simulink model "atrias_boom_nmSt_kinSw_v3"  (R2015a)
settings: Solver=ode23t  StartTime=0.0  StopTime=t_end  FixedStep=0.001  MaxStep=1e-3  RelTol=1e-3
InitFcn:
  | addpath('../common/')
  | colors
StartFcn:
  | tic
StopFcn:
  | %stopscript
values from neighbouring files (symbols this model uses):
  dt_a_dTrunk_boom = 5    [main_1_nmSt_kinSw.m]    (also in main_2_nmSt_kinSw_v2.m; main_3_nmSt_kinSw_v3.m; main_4_nmSt_kinSw_v4.m)
  dt_fade_boomCtrl = 2    [main_1_nmSt_kinSw.m]    (also in main_2_nmSt_kinSw_v2.m; main_3_nmSt_kinSw_v3.m; main_4_nmSt_kinSw_v4.m)
  initial_boom_yaw = 15*pi/180    (= 0.261799387799)    [main_2_nmSt_kinSw_v2.m]    (also in main_3_nmSt_kinSw_v3.m; main_4_nmSt_kinSw_v4.m)
  kd_boom_roll_Ctrl = 0    [main_1_nmSt_kinSw - Copy.m]    (also in main_1_nmSt_kinSw.m; main_2_nmSt_kinSw_v2.m; main_3_nmSt_kinSw_v3.m; main_4_nmSt_kinSw_v4.m)
  kd_boom_yaw_Ctrl = 0.1*kp_boom_yaw_Ctrl    (= 100000000)    [main_1_nmSt_kinSw - Copy.m]    (also in main_1_nmSt_kinSw.m = 1000000000; main_2_nmSt_kinSw_v2.m = 10000000; main_3_nmSt_kinSw_v3.m = 10000000; main_4_nmSt_kinSw_v4.m = 10000000)
  kd_motor = 0.90*2*sqrt(3.75*kp_motor)    [main_1_nmSt_kinSw - Copy.m]
  kinSw_alpha_start = 100*pi/180    (= 1.74532925199)    [main_1_nmSt_kinSw - Copy.m]    (also in main_1_nmSt_kinSw.m = 1.91986217719; main_2_nmSt_kinSw_v2.m = 1.83259571459; main_3_nmSt_kinSw_v3.m = 1.83259571459; main_4_nmSt_kinSw_v4.m = 1.83259571459)
  kinSw_alpha_tgt = 80*pi/180    (= 1.3962634016)    [main_1_nmSt_kinSw - Copy.m]    (also in main_1_nmSt_kinSw.m = 1.2217304764; main_2_nmSt_kinSw_v2.m = 1.2217304764; main_3_nmSt_kinSw_v3.m = 1.2217304764; main_4_nmSt_kinSw_v4.m = 1.2217304764)
  kinSw_t_start = 1.5    [main_1_nmSt_kinSw - Copy.m]    (also in main_1_nmSt_kinSw.m; main_2_nmSt_kinSw_v2.m = 0.5; main_3_nmSt_kinSw_v3.m = 0.5; main_4_nmSt_kinSw_v4.m = 0.5)
  kp_boom_roll_Ctrl = 0    [main_1_nmSt_kinSw - Copy.m]    (also in main_1_nmSt_kinSw.m; main_2_nmSt_kinSw_v2.m; main_3_nmSt_kinSw_v3.m; main_4_nmSt_kinSw_v4.m)
  kp_boom_yaw_Ctrl = 1e9    (= 1000000000)    [main_1_nmSt_kinSw - Copy.m]    (also in main_1_nmSt_kinSw.m = 10000000000; main_2_nmSt_kinSw_v2.m = 100000000; main_3_nmSt_kinSw_v3.m = 100000000; main_4_nmSt_kinSw_v4.m = 100000000)
  kp_motor = 3000    [main_1_nmSt_kinSw - Copy.m]
  max_back_bar_angle = 262.4*pi/180    (= 4.57974395723)    [main_1_nmSt_kinSw - Copy.m]
  max_front_bar_angle = 194.8*pi/180    (= 3.39990138288)    [main_1_nmSt_kinSw - Copy.m]
  min_back_bar_angle = 165.0*pi/180    (= 2.87979326579)    [main_1_nmSt_kinSw - Copy.m]
  min_front_bar_angle = 98.0*pi/180    (= 1.71042266695)    [main_1_nmSt_kinSw - Copy.m]
  poser_LLegAlp = (initial_l_leg_angle -pi/2)*180/pi    (= 105)    [main_2_nmSt_kinSw_v2.m]    (also in main_3_nmSt_kinSw_v3.m; main_4_nmSt_kinSw_v4.m)
  poser_LLegLen = initial_l_leg_length    (= 0.88)    [main_2_nmSt_kinSw_v2.m]    (also in main_3_nmSt_kinSw_v3.m; main_4_nmSt_kinSw_v4.m)
  poser_RLegAlp = (initial_r_leg_angle -pi/2)*180/pi    (= 75)    [main_2_nmSt_kinSw_v2.m]    (also in main_3_nmSt_kinSw_v3.m; main_4_nmSt_kinSw_v4.m)
  poser_RLegLen = initial_r_leg_length    (= 0.9)    [main_2_nmSt_kinSw_v2.m]    (also in main_3_nmSt_kinSw_v3.m; main_4_nmSt_kinSw_v4.m)
  tEnd_boomCtrl = t_end    (= 20)    [main_1_nmSt_kinSw - Copy.m]    (also in main_1_nmSt_kinSw.m = 3; main_2_nmSt_kinSw_v2.m = 7.5; main_3_nmSt_kinSw_v3.m = 7.5; main_4_nmSt_kinSw_v4.m = 7.5)
  tStart_boomCtrl = 1    [main_1_nmSt_kinSw - Copy.m]    (also in main_1_nmSt_kinSw.m = 0; main_2_nmSt_kinSw_v2.m = 0.5; main_3_nmSt_kinSw_v3.m = 0.5; main_4_nmSt_kinSw_v4.m = 0.5)
  tune_kinSw_alpha_start = kinSw_alpha_start*180/pi    (= 105)    [main_2_nmSt_kinSw_v2.m]    (also in main_3_nmSt_kinSw_v3.m; main_4_nmSt_kinSw_v4.m)
  tune_kinSw_alpha_tgt = kinSw_alpha_tgt*180/pi    (= 70)    [main_2_nmSt_kinSw_v2.m]    (also in main_3_nmSt_kinSw_v3.m; main_4_nmSt_kinSw_v4.m)
  tune_kinSw_len_min = kinSw_lclr    (= 0.7)    [main_2_nmSt_kinSw_v2.m]    (also in main_3_nmSt_kinSw_v3.m = 0.6)
  tune_kinSw_len_tgt = kinSw_len_tgt    (= 0.9)    [main_2_nmSt_kinSw_v2.m]    (also in main_3_nmSt_kinSw_v3.m)
  tune_M1_G = St_FGain_VAS*FmaxVAS    [main_2_nmSt_kinSw_v2.m]    (also in main_3_nmSt_kinSw_v3.m; main_4_nmSt_kinSw_v4.m)
  tune_M3_0 = CtrlPar_theta0*180/pi    [main_2_nmSt_kinSw_v2.m]    (also in main_3_nmSt_kinSw_v3.m; main_4_nmSt_kinSw_v4.m)
  tune_M3_D = St_GainDTh_HFL    [main_2_nmSt_kinSw_v2.m]    (also in main_3_nmSt_kinSw_v3.m; main_4_nmSt_kinSw_v4.m)
  tune_M3_P = St_GainTh_HFL    [main_2_nmSt_kinSw_v2.m]    (also in main_3_nmSt_kinSw_v3.m; main_4_nmSt_kinSw_v4.m)
  tune_M4_G = 1    [main_3_nmSt_kinSw_v3.m]    (also in main_4_nmSt_kinSw_v4.m)
  v_dTrunk_boom = 1.3    [main_1_nmSt_kinSw.m]    (also in main_2_nmSt_kinSw_v2.m; main_3_nmSt_kinSw_v3.m; main_4_nmSt_kinSw_v4.m)
undefined symbols (not defined in the file or in its folder): A1_notch_f1, A2_notch_f1, A_lpf_dtau, A_lpf_velocity, ankle_stiffness, B1_lpf_dtau, B1_lpf_velocity, B1_notch_f1, B2_lpf_dtau, B2_lpf_velocity, B2_notch_f1, b_hmotor, b_leg_spring, b_rotor, base_color_d, boom_color_d, boom_mount_to_center_diagonal, breakaway_friction, c_jointstop, contactThr, coulomb_friction, d_com, delta_phi_max, delta_phi_max_buffer, delta_phi_max_dropoff, delta_phi_min, fblink_color_d, floor_color_d, FmaxBFSH, FmaxGLU, FmaxHAM, FmaxHFL, FmaxRF, FmaxVAS, foot_color_d, FPCtrlPar, friction_linear_zone, g, gain_nodes_sea_torque, HIP_MTR_MAX_CONT_TORQUE, HIP_MTR_MAX_TORQUE, hshaft_color_d, initial_boom_pitch, initial_boom_roll, initial_hip_roll, initial_winch_angle, j_motor, k_gn, k_gt, k_leg_spring, K_notch_f1, k_phi, k_sea, Kb_leg, kd_lateral, kd_shin_max, kd_shin_min, kd_splay_max, kd_splay_min, kd_thigh_max ... (+186)
libraries: sm_lib x210, nesl_utility x140, simulink x65, simulink_extras x32, fl_lib x16, mblibv1 x2, commnoisgen2 x1
(part 6 of 17)

== system atrias_boom_nmSt_kinSw_v3/Mechanical System Layer/Ground Contact Models/flat ground (LHeel) ==
  Cnt : Inport
  Constant : Constant  Value=0
  Constant1 : Constant  Value=[0 0 1]
  Mux4 : Mux  Inputs=5
  Selector25 : Selector  InputPortWidth=3
  Selector26 : Selector  InputPortWidth=7  Indices=[1 2 3 6 4 5 7]
  Selector27 : Selector  InputPortWidth=3  Indices=3
  Env : Outport
  wires:
  Mux4/1 -> Selector26/1
  Constant1/1 -> Mux4/3
  Cnt/1 -> Selector27/1, Selector25/1
  Selector27/1 -> Mux4/4
  Constant/1 -> Mux4/5, Mux4/1
  Selector25/1 -> Mux4/2
  Selector26/1 -> Env/1

== system atrias_boom_nmSt_kinSw_v3/Mechanical System Layer/Ground Contact Models/flat ground (RBall) ==
  Cnt : Inport
  Constant : Constant  Value=0
  Constant1 : Constant  Value=[0 0 1]
  Mux4 : Mux  Inputs=5
  Selector25 : Selector  InputPortWidth=3
  Selector26 : Selector  InputPortWidth=7  Indices=[1 2 3 6 4 5 7]
  Selector27 : Selector  InputPortWidth=3  Indices=3
  Env : Outport
  wires:
  Mux4/1 -> Selector26/1
  Constant1/1 -> Mux4/3
  Cnt/1 -> Selector27/1, Selector25/1
  Selector27/1 -> Mux4/4
  Constant/1 -> Mux4/5, Mux4/1
  Selector25/1 -> Mux4/2
  Selector26/1 -> Env/1

== system atrias_boom_nmSt_kinSw_v3/Mechanical System Layer/Ground Contact Models/flat ground (RHeel) ==
  Cnt : Inport
  Constant : Constant  Value=0
  Constant1 : Constant  Value=[0 0 1]
  Mux4 : Mux  Inputs=5
  Selector25 : Selector  InputPortWidth=3
  Selector26 : Selector  InputPortWidth=7  Indices=[1 2 3 6 4 5 7]
  Selector27 : Selector  InputPortWidth=3  Indices=3
  Env : Outport
  wires:
  Mux4/1 -> Selector26/1
  Constant1/1 -> Mux4/3
  Cnt/1 -> Selector27/1, Selector25/1
  Selector27/1 -> Mux4/4
  Constant/1 -> Mux4/5, Mux4/1
  Selector25/1 -> Mux4/2
  Selector26/1 -> Env/1

== system atrias_boom_nmSt_kinSw_v3/Mechanical System Layer/L Hip Shaft/Frame Data ==
  Kinematic Data : ToWorkspace  VariableName=l_hip_out  SampleTime=output_sample_time
      settings: Save2DSignal=2-D array (concatenate along first dimension)
  Mux : Mux
  PS-Simulink Converter{,1..3} (4 alike) : nesl_utility/PS-Simulink Converter  PhysicalDomain=network_engine_domain  SubClassName=ps_output  LeftPortType=input  RightPortType=output  PseudoPeriodic=off  Frequencies=[]  Unit=1  AffineConversion=off
  Transform Sensor : sm_lib/Frames and Transforms/Transform Sensor  MeasurementFrame=World  SenseAngle=off  SenseAxis=off  SenseAngle1=off  SenseAngle2=off  SenseAngle3=off  SenseQ=on  SenseR=off  SenseOmegaX=off  SenseOmegaY=off  SenseOmegaZ=off  SenseOmega1=off  SenseOmega2=off  SenseOmega3=off  SenseQDot=off  SenseRDot=off  SenseAlphaX=off  SenseAlphaY=off  SenseAlphaZ=off  SenseAlpha1=off  SenseAlpha2=off  SenseAlpha3=off  SenseQDDot=off  SenseRDDot=off  SenseX=on  SenseY=on  SenseZ=on  SenseRad=off  SenseAzim=off  SenseDist=off  SenseInc=off  SenseXDot=off  SenseYDot=off  SenseZDot=off  SenseRadDot=off  SenseAzimDot=off  SenseDistDot=off  SenseIncDot=off  SenseXDDot=off  SenseYDDot=off  SenseZDDot=off  SenseRadDDot=off  SenseAzimDDot=off  SenseDistDDot=off  SenseIncDDot=off  BlockFunction=simmechanics.library.frames_transforms.transform_sensor
  World Frame : sm_lib/Frames and Transforms/World Frame  BlockFunction=simmechanics.library.frames_transforms.world_frame
  Frame : PMIOPort  Port=1  Side=Left
  wires:
  Mux/1 -> Kinematic Data/1
  PS-Simulink Converter/1 -> Mux/1
  PS-Simulink Converter1/1 -> Mux/2
  PS-Simulink Converter2/1 -> Mux/3
  PS-Simulink Converter3/1 -> Mux/4
  connections:
  PS-Simulink Converter3/LConn1 -- Transform Sensor/RConn5
  PS-Simulink Converter2/LConn1 -- Transform Sensor/RConn4
  PS-Simulink Converter1/LConn1 -- Transform Sensor/RConn3
  PS-Simulink Converter/LConn1 -- Transform Sensor/RConn2
  Transform Sensor/RConn1 -- Frame/RConn1
  Transform Sensor/LConn1 -- World Frame/RConn1

== system atrias_boom_nmSt_kinSw_v3/Mechanical System Layer/L Leg/Angle Range Map ==
  "[-pi, pi]" : Inport
  Constant : Constant  Value=2*pi
  Sum3 : Sum  Inputs=|++
  Switch : Switch  ZeroCross=off
  "[0,2*pi]" : Outport
  wires:
  "[-pi, pi]"/1 -> Sum3/1, Switch/1, Switch/2
  Sum3/1 -> Switch/3
  Constant/1 -> Sum3/2
  Switch/1 -> "[0,2*pi]"/1

== system atrias_boom_nmSt_kinSw_v3/Mechanical System Layer/L Leg/Angle Range Map1 ==
  "[-pi, pi]" : Inport
  Constant : Constant  Value=2*pi
  Sum3 : Sum  Inputs=|++
  Switch : Switch  ZeroCross=off
  "[0,2*pi]" : Outport
  wires:
  Switch/1 -> "[0,2*pi]"/1
  Constant/1 -> Sum3/2
  Sum3/1 -> Switch/3
  "[-pi, pi]"/1 -> Switch/2, Switch/1, Sum3/1

== system atrias_boom_nmSt_kinSw_v3/Mechanical System Layer/L Leg/Four Bar Link ==
  CS1 to CS2 : sm_lib/Frames and Transforms/Rigid Transform  TranslationMethod=Cartesian  TranslationLengthUnit=m  TranslationStandardAxis=+Z  TranslationStandardOffset=0  TranslationCartesianOffset=[0 -l_seg 0]  TranslationROffset=0  TranslationROffsetUnits=m  TranslationZOffset=0  TranslationZOffsetUnits=m  TranslationThetaOffset=0  TranslationThetaOffsetUnits=deg  RotationMethod=None  RotationAngleUnits=deg  RotationStandardAxis=+Z  RotationAngle=0  RotationArbitraryAxis=[0 0 1]  FollAlignAxisA=+X  BaseAlignAxisA=+Y  FollAlignAxisB=+Y  BaseAlignAxisB=+Z  RotationMatrix=[1 0 0; 0 1 0; 0 0 1]  BlockFunction=simmechanics.library.frames_transforms.rigid_transform
  Frame Data : Subsystem
  Solid : sm_lib/Body Elements/Solid  InertiaType=Custom  Mass=m_fblink  MassUnits=kg  CenterOfMass=com_fblink  CenterOfMassUnits=m  MomentsOfInertia=i_fblink_moments  MomentsOfInertiaUnits=kg*m^2  ProductsOfInertia=i_fblink_products  ProductsOfInertiaUnits=kg*m^2  DensityBased=on  Density=1000  DensityUnits=kg/(m^3)  GraphicType=FromGeometry  MarkerShape=Sphere  MarkerSize=10  MarkerSizeUnits=m  GraphicVisPropType=AdvancedVisualProperties  GraphicDiffuseColor=fblink_color_d  GraphicSpecularColor=[0.5 0.5 0.5 1.0]  GraphicAmbientColor=[fblink_color_d*0.5 1.0]  GraphicEmissiveColor=[0.0 0.0 0.0 1.0]  GraphicShininess=128  GraphicOpacity=1.0  GeometryShape=FromFile  RectangleSize=[1 1]  RectangleSizeUnits=m  BrickDimensions=[0.1 l_seg 0.1]  BrickDimensionUnits=m  CylinderRadius=l_rad  CylinderRadiusUnits=m  CylinderLength=l_seg  CylinderLengthUnits=m  SphereRadius=1  SphereRadiusUnits=m  EllipsoidRadii=[1 1 1]  EllipsoidRadiiUnits=m  ExtrusionCrossSection=[1 1; -1 1; -1 -1; 1 -1]  ExtrusionCrossSectionUnits=m  ExtrusionLength=1  ExtrusionLengthUnits=m  PolygonNumSides=3  PolygonOuterRadius=1  PolygonOuterRadiusUnits=m  ExtGeomFileType=STL  ExtGeomFileName=../models/four_bar_link.stl  ExtGeomFileUnits=m  RevolutionCrossSection=[1 1; 1 -1; 2 -1; 2 1]  RevolutionCrossSectionUnits=m  RevolutionExtent=Full  RevolutionAngle=180  RevolutionAngleUnits=deg  BlockFunction=simmechanics.library.body_elements.solid
  CS1 : PMIOPort  Port=1  Side=Left
  CS2 : PMIOPort  Port=2  Side=Right
  connections:
  CS2/RConn1 -- CS1 to CS2/RConn1
  Solid/RConn1 -- CS1/RConn1 -- Frame Data/LConn1 -- CS1 to CS2/LConn1

== system atrias_boom_nmSt_kinSw_v3/Mechanical System Layer/L Leg/Lower Leg ==
  CS1 to CS2 : sm_lib/Frames and Transforms/Rigid Transform  TranslationMethod=Cartesian  TranslationLengthUnit=m  TranslationStandardAxis=+Z  TranslationStandardOffset=0  TranslationCartesianOffset=[0 -lowerleg_12 0]  TranslationROffset=0  TranslationROffsetUnits=m  TranslationZOffset=0  TranslationZOffsetUnits=m  TranslationThetaOffset=0  TranslationThetaOffsetUnits=deg  RotationMethod=None  RotationAngleUnits=deg  RotationStandardAxis=+Z  RotationAngle=0  RotationArbitraryAxis=[0 0 1]  FollAlignAxisA=+X  BaseAlignAxisA=+Y  FollAlignAxisB=+Y  BaseAlignAxisB=+Z  RotationMatrix=[1 0 0; 0 1 0; 0 0 1]  BlockFunction=simmechanics.library.frames_transforms.rigid_transform
  CS1 to CS3 : sm_lib/Frames and Transforms/Rigid Transform  TranslationMethod=Cartesian  TranslationLengthUnit=m  TranslationStandardAxis=+Z  TranslationStandardOffset=0  TranslationCartesianOffset=[0 -l_seg 0]  TranslationROffset=0  TranslationROffsetUnits=m  TranslationZOffset=0  TranslationZOffsetUnits=m  TranslationThetaOffset=0  TranslationThetaOffsetUnits=deg  RotationMethod=None  RotationAngleUnits=deg  RotationStandardAxis=+Z  RotationAngle=0  RotationArbitraryAxis=[0 0 1]  FollAlignAxisA=+X  BaseAlignAxisA=+Y  FollAlignAxisB=+Y  BaseAlignAxisB=+Z  RotationMatrix=[1 0 0; 0 1 0; 0 0 1]  BlockFunction=simmechanics.library.frames_transforms.rigid_transform
  Frame Data : Subsystem
  Solid : sm_lib/Body Elements/Solid  InertiaType=Custom  Mass=m_lowerleg  MassUnits=kg  CenterOfMass=com_lowerleg  CenterOfMassUnits=m  MomentsOfInertia=i_lowerleg_moments  MomentsOfInertiaUnits=kg*m^2  ProductsOfInertia=i_lowerleg_products  ProductsOfInertiaUnits=kg*m^2  DensityBased=on  Density=1000  DensityUnits=kg/(m^3)  GraphicType=FromGeometry  MarkerShape=Sphere  MarkerSize=10  MarkerSizeUnits=m  GraphicVisPropType=AdvancedVisualProperties  GraphicDiffuseColor=lowerleg_color_d  GraphicSpecularColor=[0.5 0.5 0.5 1.0]  GraphicAmbientColor=[lowerleg_color_d*0.5 1.0]  GraphicEmissiveColor=[0.0 0.0 0.0 1.0]  GraphicShininess=128  GraphicOpacity=1.0  GeometryShape=FromFile  RectangleSize=[1 1]  RectangleSizeUnits=m  BrickDimensions=[0.1 l_seg 0.1]  BrickDimensionUnits=m  CylinderRadius=l_rad  CylinderRadiusUnits=m  CylinderLength=l_seg  CylinderLengthUnits=m  SphereRadius=1  SphereRadiusUnits=m  EllipsoidRadii=[1 1 1]  EllipsoidRadiiUnits=m  ExtrusionCrossSection=[1 1; -1 1; -1 -1; 1 -1]  ExtrusionCrossSectionUnits=m  ExtrusionLength=1  ExtrusionLengthUnits=m  PolygonNumSides=3  PolygonOuterRadius=1  PolygonOuterRadiusUnits=m  ExtGeomFileType=STL  ExtGeomFileName=../models/lower_leg.STL  ExtGeomFileUnits=m  RevolutionCrossSection=[1 1; 1 -1; 2 -1; 2 1]  RevolutionCrossSectionUnits=m  RevolutionExtent=Full  RevolutionAngle=180  RevolutionAngleUnits=deg  BlockFunction=simmechanics.library.body_elements.solid
  CS1 : PMIOPort  Port=1  Side=Left
  CS2 : PMIOPort  Port=2  Side=Right
  CS3 : PMIOPort  Port=3  Side=Right
  connections:
  CS3/RConn1 -- CS1 to CS3/RConn1
  Frame Data/LConn1 -- CS1 to CS3/LConn1 -- CS1 to CS2/LConn1 -- Solid/RConn1 -- CS1/RConn1
  CS2/RConn1 -- CS1 to CS2/RConn1

== system atrias_boom_nmSt_kinSw_v3/Mechanical System Layer/L Leg/Mechanical Limits ==
  note: Thigh-Shin Flexion Collision
  note: Thigh-Shin Collision
  note: Mechanical Limits Model
  dphi_shin : Inport
  phi_shin : Inport  Port=2
  dphi_thigh : Inport  Port=3
  phi_thigh : Inport  Port=4
  Compare To Constant5 : simulink/Logic and Bit Operations/Compare To Constant  relop=<=  const=phi_max_collision  OutDataTypeStr=boolean  ZeroCross=off
  Compare To Zero{,1..5} (6 alike) : simulink/Logic and Bit Operations/Compare To Zero  relop=<=  OutDataTypeStr=boolean  ZeroCross=off
  Constant : Constant  Value=delta_phi_min
  Constant1 : Constant  Value=phi_shin_max
  Constant2 : Constant  Value=phi_thigh_min
  Constant3 : Constant  Value=delta_phi_max
  Constant4 : Constant  Value=phi_shin_min
  Constant5 : Constant  Value=phi_thigh_max
  Enabled Subsystem : Subsystem  TreatAsAtomicUnit=on
  Gain : Gain  Gain=-1
  Gain1 : Gain  Gain=-1
  Gain2 : Gain  Gain=-1
  Logical Operator : Logic  Operator=OR  Inputs=1  AllPortsSameDT=off  OutDataTypeStr=boolean
  Mux : Mux  Inputs=6
  Shin Max Collision Model : Subsystem
  Shin Min Collision Model : Subsystem
  Stop Simulation6 : Stop
  Sum{1..3,5,7} (5 alike) : Sum  Inputs=-+|
  Sum10 : Sum  Inputs=+-|
  Sum11 : Sum  Inputs=-|+
  Sum4 : Sum  Inputs=+-|
  Sum6 : Sum  Inputs=+|-
  Sum8 : Sum  Inputs=+-|
  Sum9 : Sum  Inputs=-|+
  Thigh Max Collision Model : Subsystem
  Thigh Min Collision Model : Subsystem
  Thigh-Shin Collision Model : Subsystem
  Thigh-Shin Collision Model1 : Subsystem
  tau_shin_col : Outport
  tau_thigh_shin_col : Outport  Port=2
  tau_thigh_col : Outport  Port=3
  wires:
  Compare To Constant5/1 -> Logical Operator/1, Enabled Subsystem/1(Col_Flags)
  Sum4/1 -> Shin Max Collision Model/1(phi [rad]), Compare To Zero1/1, [col_r_shin_max]
  Sum10/1 -> [col_r_thigh_max], Compare To Zero5/1, Thigh Max Collision Model/1(phi [rad])
  Logical Operator/1 -> Enabled Subsystem/Enable, Stop Simulation6/1
  Mux/1 -> Compare To Constant5/1
  [col_r_leg_flexion] -> Mux/6
  [col_r_leg_extension] -> Mux/5
  [col_r_shin_min] -> Mux/4
  [col_r_shin_max] -> Mux/3
  [col_r_thigh_min] -> Mux/2
  [col_r_thigh_max] -> Mux/1
  Thigh Max Collision Model/1(tau_interaction[Nm]) -> Sum11/1
  Gain1/1 -> Thigh Max Collision Model/2(vphi [rad/s])
  Thigh Min Collision Model/1(tau_interaction[Nm]) -> Sum11/2
  Sum11/1 -> tau_thigh_col/1
  Compare To Zero5/1 -> Thigh Max Collision Model/Enable
  Constant5/1 -> Sum10/1
  Sum6/1 -> tau_thigh_shin_col/1
  Shin Min Collision Model/1(tau_interaction[Nm]) -> Sum9/2
  Shin Max Collision Model/1(tau_interaction[Nm]) -> Sum9/1
  Sum9/1 -> tau_shin_col/1
  dphi_shin/1 -> Shin Min Collision Model/2(vphi [rad/s]), Gain/1, Sum2/2
  Sum7/1 -> Shin Min Collision Model/1(phi [rad]), Compare To Zero4/1, [col_r_shin_min]
  Constant4/1 -> Sum7/1
  Compare To Zero4/1 -> Shin Min Collision Model/Enable
  Gain2/1 -> Thigh-Shin Collision Model1/2(vphi [rad/s])
  Thigh-Shin Collision Model1/1(tau_interaction[Nm]) -> Sum6/2
  Thigh-Shin Collision Model/1(tau_interaction[Nm]) -> Sum6/1
  Sum8/1 -> Thigh-Shin Collision Model1/1(delta_phi [rad]), Compare To Zero3/1, [col_r_leg_flexion]
  Constant3/1 -> Sum8/1
  Compare To Zero3/1 -> Thigh-Shin Collision Model1/Enable
  Compare To Zero2/1 -> Thigh Min Collision Model/Enable
  Gain/1 -> Shin Max Collision Model/2(vphi [rad/s])
  Sum5/1 -> Thigh Min Collision Model/1(phi [rad]), Compare To Zero2/1, [col_r_thigh_min]
  Constant2/1 -> Sum5/1
  dphi_thigh/1 -> Sum2/1, Gain1/1, Thigh Min Collision Model/2(vphi [rad/s])
  phi_thigh/1 -> Sum1/1, Sum5/2, Sum10/2
  Constant1/1 -> Sum4/1
  Compare To Zero1/1 -> Shin Max Collision Model/Enable
  Sum3/1 -> Thigh-Shin Collision Model/1(delta_phi [rad]), Compare To Zero/1, [col_r_leg_extension]
  Constant/1 -> Sum3/1
  Sum2/1 -> Thigh-Shin Collision Model/2(vphi [rad/s]), Gain2/1
  phi_shin/1 -> Sum4/2, Sum7/2, Sum1/2
  Sum1/1 -> Sum3/2, Sum8/2
  Compare To Zero/1 -> Thigh-Shin Collision Model/Enable

== system atrias_boom_nmSt_kinSw_v3/Mechanical System Layer/L Leg/Shin ==
  CS1 to CS2 : sm_lib/Frames and Transforms/Rigid Transform  TranslationMethod=Cartesian  TranslationLengthUnit=m  TranslationStandardAxis=+Z  TranslationStandardOffset=0  TranslationCartesianOffset=[0 -shin_12 0]  TranslationROffset=0  TranslationROffsetUnits=m  TranslationZOffset=0  TranslationZOffsetUnits=m  TranslationThetaOffset=0  TranslationThetaOffsetUnits=deg  RotationMethod=None  RotationAngleUnits=deg  RotationStandardAxis=+Z  RotationAngle=0  RotationArbitraryAxis=[0 0 1]  FollAlignAxisA=+X  BaseAlignAxisA=+Y  FollAlignAxisB=+Y  BaseAlignAxisB=+Z  RotationMatrix=[1 0 0; 0 1 0; 0 0 1]  BlockFunction=simmechanics.library.frames_transforms.rigid_transform
  Frame Data : Subsystem
  Solid : sm_lib/Body Elements/Solid  InertiaType=Custom  Mass=m_shin  MassUnits=kg  CenterOfMass=com_shin  CenterOfMassUnits=m  MomentsOfInertia=i_shin_moments  MomentsOfInertiaUnits=kg*m^2  ProductsOfInertia=i_shin_products  ProductsOfInertiaUnits=kg*m^2  DensityBased=on  Density=1000  DensityUnits=kg/(m^3)  GraphicType=FromGeometry  MarkerShape=Sphere  MarkerSize=10  MarkerSizeUnits=m  GraphicVisPropType=AdvancedVisualProperties  GraphicDiffuseColor=shin_color_d  GraphicSpecularColor=[0.5 0.5 0.5 1.0]  GraphicAmbientColor=[shin_color_d*0.5 1.0]  GraphicEmissiveColor=[0.0 0.0 0.0 1.0]  GraphicShininess=128  GraphicOpacity=1.0  GeometryShape=FromFile  RectangleSize=[1 1]  RectangleSizeUnits=m  BrickDimensions=[1 1 1]  BrickDimensionUnits=m  CylinderRadius=l_rad  CylinderRadiusUnits=m  CylinderLength=l_seg  CylinderLengthUnits=m  SphereRadius=1  SphereRadiusUnits=m  EllipsoidRadii=[1 1 1]  EllipsoidRadiiUnits=m  ExtrusionCrossSection=[1 1; -1 1; -1 -1; 1 -1]  ExtrusionCrossSectionUnits=m  ExtrusionLength=1  ExtrusionLengthUnits=m  PolygonNumSides=3  PolygonOuterRadius=1  PolygonOuterRadiusUnits=m  ExtGeomFileType=STL  ExtGeomFileName=../models/shin.STL  ExtGeomFileUnits=m  RevolutionCrossSection=[1 1; 1 -1; 2 -1; 2 1]  RevolutionCrossSectionUnits=m  RevolutionExtent=Full  RevolutionAngle=180  RevolutionAngleUnits=deg  BlockFunction=simmechanics.library.body_elements.solid
  CS1 : PMIOPort  Port=1  Side=Left
  CS2 : PMIOPort  Port=2  Side=Right
  connections:
  CS1 to CS2/LConn1 -- CS1/RConn1 -- Frame Data/LConn1 -- Solid/RConn1
  CS2/RConn1 -- CS1 to CS2/RConn1

== system atrias_boom_nmSt_kinSw_v3/Mechanical System Layer/L Leg/Shin SEA ==
  note: Shin SEA Mechanics
  Shin Gear Torque [Nm] : Inport
  Shin Joint [rad rad/s] : Inport  Port=2
  Demux : Demux  Outputs=2
  Gain : Gain  Gain=k_leg_spring
  Gain1 : Gain  Gain=b_leg_spring
  Initial Gear Angle : Constant  Value=shin_initial_l
  Inverse Gear Ratio2 : Gain  Gain=1/N
  Inverse Gear Ratio3 : Gain  Gain=Kt_leg
  Inverse Gear Ratio4 : Gain  Gain=1/Kt_leg
  Motor Efficiency : Gain  Gain=mu_motor
  Motor Controller : Subsystem  Commented=on
  Motor Electromagnetism : Subsystem  Commented=on
  Rotor Damping : Gain  Gain=b_rotor
  Rotor and Gearing : Subsystem
  Sum : Sum  Inputs=++|
  Sum2 : Sum  Inputs=+|-
  Sum3 : Sum  Inputs=|+-
  Sum4 : Sum  Inputs=+|-
  Sum5 : Sum  Inputs=|++
  Torque Limiter (outside) 2 : Saturate  UpperLimit=LEG_MTR_MAX_TORQUE  LowerLimit=-LEG_MTR_MAX_TORQUE  ZeroCross=off
      settings: AttributesFormatString=Hi: %<UpperLimit>\nLo: %<LowerLimit>
  Rotor Joint Conn : PMIOPort  Port=1  Side=Left
  Shin Joint Torque [Nm] : Outport
  Shin Gear [rad] : Outport  Port=2
  wires:
  Sum2/1 -> Gain/1
  Sum5/1 -> Rotor and Gearing/2(Spring Torque [Nm]), Shin Joint Torque [Nm]/1
  Sum3/1 -> Motor Efficiency/1
  Rotor Damping/1 -> Sum3/2
  Gain/1 -> Sum5/1  "tau_load"
  Gain1/1 -> Sum5/2
  Sum4/1 -> Gain1/1
  Shin Joint [rad rad/s]/1 -> Demux/1
  Demux/1 -> Sum2/2
  Demux/2 -> Sum4/2
  Inverse Gear Ratio3/1 -> Sum3/1
  Initial Gear Angle/1 -> Sum/1
  Sum/1 -> Shin Gear [rad]/1, Sum2/1
  Rotor and Gearing/1(Gearhead Position [rad]) -> Sum/2
  Rotor and Gearing/2(Gearhead Velocity [rad/s]) -> Sum4/1
  Motor Efficiency/1 -> Rotor and Gearing/1(Rotor Torque [Nm])
  Inverse Gear Ratio4/1 -> Inverse Gear Ratio3/1
  Motor Controller/1(Voltage [V]) -> Motor Electromagnetism/1(Voltage [V])
  Motor Electromagnetism/1(Current [A]) -> Motor Controller/2(Measured Current [A])
  Shin Gear Torque [Nm]/1 -> Torque Limiter (outside) 2/1
  Inverse Gear Ratio2/1 -> Inverse Gear Ratio4/1
  Rotor and Gearing/3(Rotor Velocity [rad/s]) -> Rotor Damping/1
  Torque Limiter (outside) 2/1 -> Inverse Gear Ratio2/1
  connections:
  Rotor and Gearing/LConn1 -- Rotor Joint Conn/RConn1

== system atrias_boom_nmSt_kinSw_v3/Mechanical System Layer/L Leg/Thigh ==
  CS1 to CS2 : sm_lib/Frames and Transforms/Rigid Transform  TranslationMethod=Cartesian  TranslationLengthUnit=m  TranslationStandardAxis=+Z  TranslationStandardOffset=0  TranslationCartesianOffset=[0 -l_seg 0]  TranslationROffset=0  TranslationROffsetUnits=m  TranslationZOffset=0  TranslationZOffsetUnits=m  TranslationThetaOffset=0  TranslationThetaOffsetUnits=deg  RotationMethod=None  RotationAngleUnits=deg  RotationStandardAxis=+Z  RotationAngle=0  RotationArbitraryAxis=[0 0 1]  FollAlignAxisA=+X  BaseAlignAxisA=+Y  FollAlignAxisB=+Y  BaseAlignAxisB=+Z  RotationMatrix=[1 0 0; 0 1 0; 0 0 1]  BlockFunction=simmechanics.library.frames_transforms.rigid_transform
  Frame Data : Subsystem
  Solid : sm_lib/Body Elements/Solid  InertiaType=Custom  Mass=m_thigh  MassUnits=kg  CenterOfMass=com_thigh  CenterOfMassUnits=m  MomentsOfInertia=i_thigh_moments  MomentsOfInertiaUnits=kg*m^2  ProductsOfInertia=i_thigh_products  ProductsOfInertiaUnits=kg*m^2  DensityBased=on  Density=1000  DensityUnits=kg/(m^3)  GraphicType=FromGeometry  MarkerShape=Sphere  MarkerSize=10  MarkerSizeUnits=m  GraphicVisPropType=AdvancedVisualProperties  GraphicDiffuseColor=thigh_color_d  GraphicSpecularColor=[0.5 0.5 0.5 1.0]  GraphicAmbientColor=[thigh_color_d*0.5 1.0]  GraphicEmissiveColor=[0.0 0.0 0.0 1.0]  GraphicShininess=128  GraphicOpacity=1.0  GeometryShape=FromFile  RectangleSize=[1 1]  RectangleSizeUnits=m  BrickDimensions=[1 1 1]  BrickDimensionUnits=m  CylinderRadius=l_rad  CylinderRadiusUnits=m  CylinderLength=l_seg  CylinderLengthUnits=m  SphereRadius=1  SphereRadiusUnits=m  EllipsoidRadii=[1 1 1]  EllipsoidRadiiUnits=m  ExtrusionCrossSection=[1 1; -1 1; -1 -1; 1 -1]  ExtrusionCrossSectionUnits=m  ExtrusionLength=1  ExtrusionLengthUnits=m  PolygonNumSides=3  PolygonOuterRadius=1  PolygonOuterRadiusUnits=m  ExtGeomFileType=STL  ExtGeomFileName=../models/thigh.STL  ExtGeomFileUnits=m  RevolutionCrossSection=[1 1; 1 -1; 2 -1; 2 1]  RevolutionCrossSectionUnits=m  RevolutionExtent=Full  RevolutionAngle=180  RevolutionAngleUnits=deg  BlockFunction=simmechanics.library.body_elements.solid
  CS1 : PMIOPort  Port=1  Side=Left
  CS2 : PMIOPort  Port=2  Side=Right
  connections:
  CS2/RConn1 -- CS1 to CS2/RConn1
  CS1 to CS2/LConn1 -- Solid/RConn1 -- Frame Data/LConn1 -- CS1/RConn1

== system atrias_boom_nmSt_kinSw_v3/Mechanical System Layer/L Leg/Thigh SEA ==
  note: Thigh SEA Mechanics
  Thigh Gear Torque [Nm] : Inport
  Thigh Joint [rad rad/s] : Inport  Port=2
  Continuous Angle : mblibv1/Utilities/Continuous Angle  rad=rad  rads=rad/s
  Demux : Demux  Outputs=2
  Gain : Gain  Gain=k_leg_spring
  Gain1 : Gain  Gain=b_leg_spring
  Initial Gear Angle : Constant  Value=thigh_initial_l
  Inverse Gear Ratio1 : Gain  Gain=1/N
  Inverse Gear Ratio2 : Gain  Gain=Kt_leg
  Inverse Gear Ratio3 : Gain  Gain=1/Kt_leg
  Motor Efficiency : Gain  Gain=mu_motor
  Motor Controller : Subsystem  Commented=on
  Motor Electromagnetism : Subsystem  Commented=on
  Rotor Damping : Gain  Gain=b_rotor
  Rotor and Gearing : Subsystem
  Sum : Sum  Inputs=++|
  Sum2 : Sum  Inputs=+|-
  Sum3 : Sum  Inputs=|+-
  Sum4 : Sum  Inputs=+|-
  Sum5 : Sum  Inputs=|++
  Torque Limiter (outside) 2 : Saturate  UpperLimit=LEG_MTR_MAX_TORQUE  LowerLimit=-LEG_MTR_MAX_TORQUE  ZeroCross=off
      settings: AttributesFormatString=Hi: %<UpperLimit>\nLo: %<LowerLimit>
  Rotor Joint Conn : PMIOPort  Port=1  Side=Left
  Thigh Joint Torque [Nm] : Outport
  Thigh Gear [rad] : Outport  Port=2
  wires:
  Sum2/1 -> Gain/1
  Sum3/1 -> Motor Efficiency/1
  Rotor Damping/1 -> Sum3/2
  Gain/1 -> Sum5/1  "tau_load"
  Gain1/1 -> Sum5/2
  Sum4/1 -> Gain1/1
  Thigh Joint [rad rad/s]/1 -> Demux/1
  Demux/1 -> Sum2/2
  Demux/2 -> Sum4/2
  Inverse Gear Ratio3/1 -> Inverse Gear Ratio2/1
  Inverse Gear Ratio2/1 -> Sum3/1
  Initial Gear Angle/1 -> Sum/1
  Sum/1 -> Thigh Gear [rad]/1, Sum2/1
  Continuous Angle/1 -> Sum/2
  Rotor and Gearing/2(Gearhead Velocity [rad/s]) -> Sum4/1, Continuous Angle/2
  Rotor and Gearing/1(Gearhead Position [rad]) -> Continuous Angle/1
  Motor Controller/1(Voltage [V]) -> Motor Electromagnetism/1(Voltage [V])
  Motor Electromagnetism/1(Current [A]) -> Motor Controller/2(Measured Current [A])
  Thigh Gear Torque [Nm]/1 -> Torque Limiter (outside) 2/1
  Inverse Gear Ratio1/1 -> Inverse Gear Ratio3/1
  Sum5/1 -> Rotor and Gearing/2(Spring Torque [Nm]), Thigh Joint Torque [Nm]/1
  Motor Efficiency/1 -> Rotor and Gearing/1(Rotor Torque [Nm])
  Rotor and Gearing/3(Rotor Velocity [rad/s]) -> Rotor Damping/1
  Torque Limiter (outside) 2/1 -> Inverse Gear Ratio1/1
  connections:
  Rotor and Gearing/LConn1 -- Rotor Joint Conn/RConn1

== system atrias_boom_nmSt_kinSw_v3/Mechanical System Layer/Left Hip Roll Joint/Mechanical Limits  ==
  vphi : Inport
  phi : Inport  Port=2
  Compare To Constant5 : simulink/Logic and Bit Operations/Compare To Constant  relop=<=  const=phi_max_collision  OutDataTypeStr=boolean  ZeroCross=off
  Compare To Zero1 : simulink/Logic and Bit Operations/Compare To Zero  relop=<=  OutDataTypeStr=boolean  ZeroCross=off
  Compare To Zero2 : simulink/Logic and Bit Operations/Compare To Zero  relop=<=  OutDataTypeStr=boolean  ZeroCross=off
  Constant1 : Constant  Value=phi_roll_min
  Constant2 : Constant  Value=phi_roll_max
  Enabled Subsystem : Subsystem  TreatAsAtomicUnit=on
  Gain2 : Gain  Gain=-1
  Logical Operator : Logic  Operator=OR  Inputs=1  AllPortsSameDT=off  OutDataTypeStr=boolean
  Mux : Mux  Inputs=2
  Roll Max Collision Model : Subsystem
  Roll Min Collision Model : Subsystem
  Stop Simulation6 : Stop
  Sum1 : Sum  Inputs=-+|
  Sum11 : Sum  Inputs=-|+
  Sum5 : Sum  Inputs=+-|
  tau_reaction : Outport
  wires:
  Gain2/1 -> Roll Max Collision Model/2(vphi [rad/s])
  vphi/1 -> Gain2/1, Roll Min Collision Model/2(vphi [rad/s])
  Roll Max Collision Model/1(tau_interaction[Nm]) -> Sum11/1
  Compare To Zero2/1 -> Roll Max Collision Model/Enable
  Sum5/1 -> Roll Max Collision Model/1(phi [rad]), Compare To Zero2/1, [col_hip_max]
  Constant2/1 -> Sum5/1
  Compare To Constant5/1 -> Logical Operator/1, Enabled Subsystem/1(Col_Flags)
  Constant1/1 -> Sum1/1
  Sum11/1 -> tau_reaction/1
  [col_hip_min] -> Mux/2
  Mux/1 -> Compare To Constant5/1
  [col_hip_max] -> Mux/1
  Logical Operator/1 -> Stop Simulation6/1, Enabled Subsystem/Enable
  phi/1 -> Sum5/2, Sum1/2
  Compare To Zero1/1 -> Roll Min Collision Model/Enable
  Roll Min Collision Model/1(tau_interaction[Nm]) -> Sum11/2
  Sum1/1 -> Roll Min Collision Model/1(phi [rad]), Compare To Zero1/1, [col_hip_min]

== system atrias_boom_nmSt_kinSw_v3/Mechanical System Layer/R Hip Shaft/Frame Data ==
  Kinematic Data : ToWorkspace  VariableName=r_hip_out  SampleTime=output_sample_time
      settings: Save2DSignal=2-D array (concatenate along first dimension)
  Mux : Mux
  PS-Simulink Converter{,1..3} (4 alike) : nesl_utility/PS-Simulink Converter  PhysicalDomain=network_engine_domain  SubClassName=ps_output  LeftPortType=input  RightPortType=output  PseudoPeriodic=off  Frequencies=[]  Unit=1  AffineConversion=off
  Transform Sensor : sm_lib/Frames and Transforms/Transform Sensor  MeasurementFrame=World  SenseAngle=off  SenseAxis=off  SenseAngle1=off  SenseAngle2=off  SenseAngle3=off  SenseQ=on  SenseR=off  SenseOmegaX=off  SenseOmegaY=off  SenseOmegaZ=off  SenseOmega1=off  SenseOmega2=off  SenseOmega3=off  SenseQDot=off  SenseRDot=off  SenseAlphaX=off  SenseAlphaY=off  SenseAlphaZ=off  SenseAlpha1=off  SenseAlpha2=off  SenseAlpha3=off  SenseQDDot=off  SenseRDDot=off  SenseX=on  SenseY=on  SenseZ=on  SenseRad=off  SenseAzim=off  SenseDist=off  SenseInc=off  SenseXDot=off  SenseYDot=off  SenseZDot=off  SenseRadDot=off  SenseAzimDot=off  SenseDistDot=off  SenseIncDot=off  SenseXDDot=off  SenseYDDot=off  SenseZDDot=off  SenseRadDDot=off  SenseAzimDDot=off  SenseDistDDot=off  SenseIncDDot=off  BlockFunction=simmechanics.library.frames_transforms.transform_sensor
  World Frame : sm_lib/Frames and Transforms/World Frame  BlockFunction=simmechanics.library.frames_transforms.world_frame
  Frame : PMIOPort  Port=1  Side=Left
  wires:
  Mux/1 -> Kinematic Data/1
  PS-Simulink Converter/1 -> Mux/1
  PS-Simulink Converter1/1 -> Mux/2
  PS-Simulink Converter2/1 -> Mux/3
  PS-Simulink Converter3/1 -> Mux/4
  connections:
  PS-Simulink Converter3/LConn1 -- Transform Sensor/RConn5
  PS-Simulink Converter2/LConn1 -- Transform Sensor/RConn4
  PS-Simulink Converter1/LConn1 -- Transform Sensor/RConn3
  PS-Simulink Converter/LConn1 -- Transform Sensor/RConn2
  Transform Sensor/RConn1 -- Frame/RConn1
  Transform Sensor/LConn1 -- World Frame/RConn1

== system atrias_boom_nmSt_kinSw_v3/Mechanical System Layer/R Leg/Angle Range Map ==
  "[-pi, pi]" : Inport
  Constant : Constant  Value=2*pi
  Sum3 : Sum  Inputs=|++
  Switch : Switch  ZeroCross=off
  "[0,2*pi]" : Outport
  wires:
  "[-pi, pi]"/1 -> Sum3/1, Switch/1, Switch/2
  Sum3/1 -> Switch/3
  Constant/1 -> Sum3/2
  Switch/1 -> "[0,2*pi]"/1

== system atrias_boom_nmSt_kinSw_v3/Mechanical System Layer/R Leg/Angle Range Map1 ==
  "[-pi, pi]" : Inport
  Constant : Constant  Value=2*pi
  Sum3 : Sum  Inputs=|++
  Switch : Switch  ZeroCross=off
  "[0,2*pi]" : Outport
  wires:
  Switch/1 -> "[0,2*pi]"/1
  Constant/1 -> Sum3/2
  Sum3/1 -> Switch/3
  "[-pi, pi]"/1 -> Switch/2, Switch/1, Sum3/1

== system atrias_boom_nmSt_kinSw_v3/Mechanical System Layer/R Leg/Four Bar Link ==
  CS1 to CS2 : sm_lib/Frames and Transforms/Rigid Transform  TranslationMethod=Cartesian  TranslationLengthUnit=m  TranslationStandardAxis=+Z  TranslationStandardOffset=0  TranslationCartesianOffset=[0 -l_seg 0]  TranslationROffset=0  TranslationROffsetUnits=m  TranslationZOffset=0  TranslationZOffsetUnits=m  TranslationThetaOffset=0  TranslationThetaOffsetUnits=deg  RotationMethod=None  RotationAngleUnits=deg  RotationStandardAxis=+Z  RotationAngle=0  RotationArbitraryAxis=[0 0 1]  FollAlignAxisA=+X  BaseAlignAxisA=+Y  FollAlignAxisB=+Y  BaseAlignAxisB=+Z  RotationMatrix=[1 0 0; 0 1 0; 0 0 1]  BlockFunction=simmechanics.library.frames_transforms.rigid_transform
  Frame Data : Subsystem
  Solid : sm_lib/Body Elements/Solid  InertiaType=Custom  Mass=m_fblink  MassUnits=kg  CenterOfMass=com_fblink  CenterOfMassUnits=m  MomentsOfInertia=i_fblink_moments  MomentsOfInertiaUnits=kg*m^2  ProductsOfInertia=i_fblink_products  ProductsOfInertiaUnits=kg*m^2  DensityBased=on  Density=1000  DensityUnits=kg/(m^3)  GraphicType=FromGeometry  MarkerShape=Sphere  MarkerSize=10  MarkerSizeUnits=m  GraphicVisPropType=AdvancedVisualProperties  GraphicDiffuseColor=fblink_color_d  GraphicSpecularColor=[0.5 0.5 0.5 1.0]  GraphicAmbientColor=[fblink_color_d*0.5 1.0]  GraphicEmissiveColor=[0.0 0.0 0.0 1.0]  GraphicShininess=128  GraphicOpacity=1.0  GeometryShape=FromFile  RectangleSize=[1 1]  RectangleSizeUnits=m  BrickDimensions=[0.1 l_seg 0.1]  BrickDimensionUnits=m  CylinderRadius=l_rad  CylinderRadiusUnits=m  CylinderLength=l_seg  CylinderLengthUnits=m  SphereRadius=1  SphereRadiusUnits=m  EllipsoidRadii=[1 1 1]  EllipsoidRadiiUnits=m  ExtrusionCrossSection=[1 1; -1 1; -1 -1; 1 -1]  ExtrusionCrossSectionUnits=m  ExtrusionLength=1  ExtrusionLengthUnits=m  PolygonNumSides=3  PolygonOuterRadius=1  PolygonOuterRadiusUnits=m  ExtGeomFileType=STL  ExtGeomFileName=../models/four_bar_link.stl  ExtGeomFileUnits=m  RevolutionCrossSection=[1 1; 1 -1; 2 -1; 2 1]  RevolutionCrossSectionUnits=m  RevolutionExtent=Full  RevolutionAngle=180  RevolutionAngleUnits=deg  BlockFunction=simmechanics.library.body_elements.solid
  CS1 : PMIOPort  Port=1  Side=Left
  CS2 : PMIOPort  Port=2  Side=Right
  connections:
  CS2/RConn1 -- CS1 to CS2/RConn1
  Solid/RConn1 -- CS1/RConn1 -- Frame Data/LConn1 -- CS1 to CS2/LConn1

== system atrias_boom_nmSt_kinSw_v3/Mechanical System Layer/R Leg/Lower Leg ==
  CS1 to CS2 : sm_lib/Frames and Transforms/Rigid Transform  TranslationMethod=Cartesian  TranslationLengthUnit=m  TranslationStandardAxis=+Z  TranslationStandardOffset=0  TranslationCartesianOffset=[0 -lowerleg_12 0]  TranslationROffset=0  TranslationROffsetUnits=m  TranslationZOffset=0  TranslationZOffsetUnits=m  TranslationThetaOffset=0  TranslationThetaOffsetUnits=deg  RotationMethod=None  RotationAngleUnits=deg  RotationStandardAxis=+Z  RotationAngle=0  RotationArbitraryAxis=[0 0 1]  FollAlignAxisA=+X  BaseAlignAxisA=+Y  FollAlignAxisB=+Y  BaseAlignAxisB=+Z  RotationMatrix=[1 0 0; 0 1 0; 0 0 1]  BlockFunction=simmechanics.library.frames_transforms.rigid_transform
  CS1 to CS3 : sm_lib/Frames and Transforms/Rigid Transform  TranslationMethod=Cartesian  TranslationLengthUnit=m  TranslationStandardAxis=+Z  TranslationStandardOffset=0  TranslationCartesianOffset=[0 -l_seg 0]  TranslationROffset=0  TranslationROffsetUnits=m  TranslationZOffset=0  TranslationZOffsetUnits=m  TranslationThetaOffset=0  TranslationThetaOffsetUnits=deg  RotationMethod=None  RotationAngleUnits=deg  RotationStandardAxis=+Z  RotationAngle=0  RotationArbitraryAxis=[0 0 1]  FollAlignAxisA=+X  BaseAlignAxisA=+Y  FollAlignAxisB=+Y  BaseAlignAxisB=+Z  RotationMatrix=[1 0 0; 0 1 0; 0 0 1]  BlockFunction=simmechanics.library.frames_transforms.rigid_transform
  Frame Data : Subsystem
  Solid : sm_lib/Body Elements/Solid  InertiaType=Custom  Mass=m_lowerleg  MassUnits=kg  CenterOfMass=com_lowerleg  CenterOfMassUnits=m  MomentsOfInertia=i_lowerleg_moments  MomentsOfInertiaUnits=kg*m^2  ProductsOfInertia=i_lowerleg_products  ProductsOfInertiaUnits=kg*m^2  DensityBased=on  Density=1000  DensityUnits=kg/(m^3)  GraphicType=FromGeometry  MarkerShape=Sphere  MarkerSize=10  MarkerSizeUnits=m  GraphicVisPropType=AdvancedVisualProperties  GraphicDiffuseColor=lowerleg_color_d  GraphicSpecularColor=[0.5 0.5 0.5 1.0]  GraphicAmbientColor=[lowerleg_color_d*0.5 1.0]  GraphicEmissiveColor=[0.0 0.0 0.0 1.0]  GraphicShininess=128  GraphicOpacity=1.0  GeometryShape=FromFile  RectangleSize=[1 1]  RectangleSizeUnits=m  BrickDimensions=[0.1 l_seg 0.1]  BrickDimensionUnits=m  CylinderRadius=l_rad  CylinderRadiusUnits=m  CylinderLength=l_seg  CylinderLengthUnits=m  SphereRadius=1  SphereRadiusUnits=m  EllipsoidRadii=[1 1 1]  EllipsoidRadiiUnits=m  ExtrusionCrossSection=[1 1; -1 1; -1 -1; 1 -1]  ExtrusionCrossSectionUnits=m  ExtrusionLength=1  ExtrusionLengthUnits=m  PolygonNumSides=3  PolygonOuterRadius=1  PolygonOuterRadiusUnits=m  ExtGeomFileType=STL  ExtGeomFileName=../models/lower_leg.STL  ExtGeomFileUnits=m  RevolutionCrossSection=[1 1; 1 -1; 2 -1; 2 1]  RevolutionCrossSectionUnits=m  RevolutionExtent=Full  RevolutionAngle=180  RevolutionAngleUnits=deg  BlockFunction=simmechanics.library.body_elements.solid
  CS1 : PMIOPort  Port=1  Side=Left
  CS2 : PMIOPort  Port=2  Side=Right
  CS3 : PMIOPort  Port=3  Side=Right
  connections:
  CS3/RConn1 -- CS1 to CS3/RConn1
  CS1 to CS3/LConn1 -- CS1 to CS2/LConn1 -- Solid/RConn1 -- Frame Data/LConn1 -- CS1/RConn1
  CS2/RConn1 -- CS1 to CS2/RConn1

== system atrias_boom_nmSt_kinSw_v3/Mechanical System Layer/R Leg/Mechanical Limits ==
  note: Thigh-Shin Flexion Collision
  note: Thigh-Shin Collision
  note: Mechanical Limits Model
  dphi_shin : Inport
  phi_shin : Inport  Port=2
  dphi_thigh : Inport  Port=3
  phi_thigh : Inport  Port=4
  Compare To Constant5 : simulink/Logic and Bit Operations/Compare To Constant  relop=<=  const=phi_max_collision  OutDataTypeStr=boolean  ZeroCross=off
  Compare To Zero{,1..5} (6 alike) : simulink/Logic and Bit Operations/Compare To Zero  relop=<=  OutDataTypeStr=boolean  ZeroCross=off
  Constant : Constant  Value=delta_phi_min
  Constant1 : Constant  Value=phi_shin_max
  Constant2 : Constant  Value=phi_thigh_min
  Constant3 : Constant  Value=delta_phi_max
  Constant4 : Constant  Value=phi_shin_min
  Constant5 : Constant  Value=phi_thigh_max
  Enabled Subsystem : Subsystem  TreatAsAtomicUnit=on
  Gain : Gain  Gain=-1
  Gain1 : Gain  Gain=-1
  Gain2 : Gain  Gain=-1
  Logical Operator : Logic  Operator=OR  Inputs=1  AllPortsSameDT=off  OutDataTypeStr=boolean
  Mux : Mux  Inputs=6
  Shin Max Collision Model : Subsystem
  Shin Min Collision Model : Subsystem
  Stop Simulation6 : Stop
  Sum{1..3,5,7} (5 alike) : Sum  Inputs=-+|
  Sum10 : Sum  Inputs=+-|
  Sum11 : Sum  Inputs=-|+
  Sum4 : Sum  Inputs=+-|
  Sum6 : Sum  Inputs=+|-
  Sum8 : Sum  Inputs=+-|
  Sum9 : Sum  Inputs=-|+
  Thigh Max Collision Model : Subsystem
  Thigh Min Collision Model : Subsystem
  Thigh-Shin Collision Model : Subsystem
  Thigh-Shin Collision Model1 : Subsystem
  tau_shin_col : Outport
  tau_thigh_shin_col : Outport  Port=2
  tau_thigh_col : Outport  Port=3
  wires:
  Compare To Constant5/1 -> Logical Operator/1, Enabled Subsystem/1(Col_Flags)
  Sum4/1 -> Shin Max Collision Model/1(phi [rad]), Compare To Zero1/1, [col_r_shin_max]
  Sum10/1 -> [col_r_thigh_max], Compare To Zero5/1, Thigh Max Collision Model/1(phi [rad])
  Logical Operator/1 -> Enabled Subsystem/Enable, Stop Simulation6/1
  Mux/1 -> Compare To Constant5/1
  [col_r_leg_flexion] -> Mux/6
  [col_r_leg_extension] -> Mux/5
  [col_r_shin_min] -> Mux/4
  [col_r_shin_max] -> Mux/3
  [col_r_thigh_min] -> Mux/2
  [col_r_thigh_max] -> Mux/1
  Thigh Max Collision Model/1(tau_interaction[Nm]) -> Sum11/1
  Gain1/1 -> Thigh Max Collision Model/2(vphi [rad/s])
  Thigh Min Collision Model/1(tau_interaction[Nm]) -> Sum11/2
  Sum11/1 -> tau_thigh_col/1
  Compare To Zero5/1 -> Thigh Max Collision Model/Enable
  Constant5/1 -> Sum10/1
  Sum6/1 -> tau_thigh_shin_col/1
  Shin Min Collision Model/1(tau_interaction[Nm]) -> Sum9/2
  Shin Max Collision Model/1(tau_interaction[Nm]) -> Sum9/1
  Sum9/1 -> tau_shin_col/1
  dphi_shin/1 -> Shin Min Collision Model/2(vphi [rad/s]), Gain/1, Sum2/2
  Sum7/1 -> Shin Min Collision Model/1(phi [rad]), Compare To Zero4/1, [col_r_shin_min]
  Constant4/1 -> Sum7/1
  Compare To Zero4/1 -> Shin Min Collision Model/Enable
  Gain2/1 -> Thigh-Shin Collision Model1/2(vphi [rad/s])
  Thigh-Shin Collision Model1/1(tau_interaction[Nm]) -> Sum6/2
  Thigh-Shin Collision Model/1(tau_interaction[Nm]) -> Sum6/1
  Sum8/1 -> Thigh-Shin Collision Model1/1(delta_phi [rad]), Compare To Zero3/1, [col_r_leg_flexion]
  Constant3/1 -> Sum8/1
  Compare To Zero3/1 -> Thigh-Shin Collision Model1/Enable
  Compare To Zero2/1 -> Thigh Min Collision Model/Enable
  Gain/1 -> Shin Max Collision Model/2(vphi [rad/s])
  Sum5/1 -> Thigh Min Collision Model/1(phi [rad]), Compare To Zero2/1, [col_r_thigh_min]
  Constant2/1 -> Sum5/1
  dphi_thigh/1 -> Sum2/1, Gain1/1, Thigh Min Collision Model/2(vphi [rad/s])
  phi_thigh/1 -> Sum1/1, Sum5/2, Sum10/2
  Constant1/1 -> Sum4/1
  Compare To Zero1/1 -> Shin Max Collision Model/Enable
  Sum3/1 -> Thigh-Shin Collision Model/1(delta_phi [rad]), Compare To Zero/1, [col_r_leg_extension]
  Constant/1 -> Sum3/1
  Sum2/1 -> Thigh-Shin Collision Model/2(vphi [rad/s]), Gain2/1
  phi_shin/1 -> Sum4/2, Sum7/2, Sum1/2
  Sum1/1 -> Sum3/2, Sum8/2
  Compare To Zero/1 -> Thigh-Shin Collision Model/Enable

== system atrias_boom_nmSt_kinSw_v3/Mechanical System Layer/R Leg/Shin ==
  CS1 to CS2 : sm_lib/Frames and Transforms/Rigid Transform  TranslationMethod=Cartesian  TranslationLengthUnit=m  TranslationStandardAxis=+Z  TranslationStandardOffset=0  TranslationCartesianOffset=[0 -shin_12 0]  TranslationROffset=0  TranslationROffsetUnits=m  TranslationZOffset=0  TranslationZOffsetUnits=m  TranslationThetaOffset=0  TranslationThetaOffsetUnits=deg  RotationMethod=None  RotationAngleUnits=deg  RotationStandardAxis=+Z  RotationAngle=0  RotationArbitraryAxis=[0 0 1]  FollAlignAxisA=+X  BaseAlignAxisA=+Y  FollAlignAxisB=+Y  BaseAlignAxisB=+Z  RotationMatrix=[1 0 0; 0 1 0; 0 0 1]  BlockFunction=simmechanics.library.frames_transforms.rigid_transform
  Frame Data : Subsystem
  Solid : sm_lib/Body Elements/Solid  InertiaType=Custom  Mass=m_shin  MassUnits=kg  CenterOfMass=com_shin  CenterOfMassUnits=m  MomentsOfInertia=i_shin_moments  MomentsOfInertiaUnits=kg*m^2  ProductsOfInertia=i_shin_products  ProductsOfInertiaUnits=kg*m^2  DensityBased=on  Density=1000  DensityUnits=kg/(m^3)  GraphicType=FromGeometry  MarkerShape=Sphere  MarkerSize=10  MarkerSizeUnits=m  GraphicVisPropType=AdvancedVisualProperties  GraphicDiffuseColor=shin_color_d  GraphicSpecularColor=[0.5 0.5 0.5 1.0]  GraphicAmbientColor=[shin_color_d*0.5 1.0]  GraphicEmissiveColor=[0.0 0.0 0.0 1.0]  GraphicShininess=128  GraphicOpacity=1.0  GeometryShape=FromFile  RectangleSize=[1 1]  RectangleSizeUnits=m  BrickDimensions=[1 1 1]  BrickDimensionUnits=m  CylinderRadius=l_rad  CylinderRadiusUnits=m  CylinderLength=l_seg  CylinderLengthUnits=m  SphereRadius=1  SphereRadiusUnits=m  EllipsoidRadii=[1 1 1]  EllipsoidRadiiUnits=m  ExtrusionCrossSection=[1 1; -1 1; -1 -1; 1 -1]  ExtrusionCrossSectionUnits=m  ExtrusionLength=1  ExtrusionLengthUnits=m  PolygonNumSides=3  PolygonOuterRadius=1  PolygonOuterRadiusUnits=m  ExtGeomFileType=STL  ExtGeomFileName=../models/shin.STL  ExtGeomFileUnits=m  RevolutionCrossSection=[1 1; 1 -1; 2 -1; 2 1]  RevolutionCrossSectionUnits=m  RevolutionExtent=Full  RevolutionAngle=180  RevolutionAngleUnits=deg  BlockFunction=simmechanics.library.body_elements.solid
  CS1 : PMIOPort  Port=1  Side=Left
  CS2 : PMIOPort  Port=2  Side=Right
  connections:
  CS1 to CS2/LConn1 -- CS1/RConn1 -- Frame Data/LConn1 -- Solid/RConn1
  CS2/RConn1 -- CS1 to CS2/RConn1

== system atrias_boom_nmSt_kinSw_v3/Mechanical System Layer/R Leg/Shin SEA ==
  note: Shin SEA Mechanics
  Shin Gear Torque [Nm] : Inport
  Shin Joint [rad rad/s] : Inport  Port=2
  Demux : Demux  Outputs=2
  Gain : Gain  Gain=k_leg_spring
  Gain1 : Gain  Gain=b_leg_spring
  Initial Gear Angle : Constant  Value=shin_initial_r
  Inverse Gear Ratio2 : Gain  Gain=1/N
  Inverse Gear Ratio3 : Gain  Gain=Kt_leg
  Inverse Gear Ratio4 : Gain  Gain=1/Kt_leg
  Motor Efficiency : Gain  Gain=mu_motor
  Motor Controller : Subsystem  Commented=on
  Motor Electromagnetism : Subsystem  Commented=on
  Rotor Damping : Gain  Gain=b_rotor
  Rotor and Gearing : Subsystem
  Sum : Sum  Inputs=++|
  Sum2 : Sum  Inputs=+|-
  Sum3 : Sum  Inputs=|+-
  Sum4 : Sum  Inputs=+|-
  Sum5 : Sum  Inputs=|++
  Torque Limiter (outside) 2 : Saturate  UpperLimit=LEG_MTR_MAX_TORQUE  LowerLimit=-LEG_MTR_MAX_TORQUE  ZeroCross=off
      settings: AttributesFormatString=Hi: %<UpperLimit>\nLo: %<LowerLimit>
  Rotor Joint Conn : PMIOPort  Port=1  Side=Left
  Shin Joint Torque [Nm] : Outport
  Shin Gear [rad] : Outport  Port=2
  wires:
  Sum2/1 -> Gain/1
  Sum5/1 -> Rotor and Gearing/2(Spring Torque [Nm]), Shin Joint Torque [Nm]/1
  Sum3/1 -> Motor Efficiency/1
  Rotor Damping/1 -> Sum3/2
  Gain/1 -> Sum5/1  "tau_load"
  Gain1/1 -> Sum5/2
  Sum4/1 -> Gain1/1
  Shin Joint [rad rad/s]/1 -> Demux/1
  Demux/1 -> Sum2/2
  Demux/2 -> Sum4/2
  Inverse Gear Ratio3/1 -> Sum3/1
  Initial Gear Angle/1 -> Sum/1
  Sum/1 -> Shin Gear [rad]/1, Sum2/1
  Rotor and Gearing/1(Gearhead Position [rad]) -> Sum/2
  Rotor and Gearing/2(Gearhead Velocity [rad/s]) -> Sum4/1
  Motor Efficiency/1 -> Rotor and Gearing/1(Rotor Torque [Nm])
  Inverse Gear Ratio4/1 -> Inverse Gear Ratio3/1
  Motor Controller/1(Voltage [V]) -> Motor Electromagnetism/1(Voltage [V])
  Motor Electromagnetism/1(Current [A]) -> Motor Controller/2(Measured Current [A])
  Shin Gear Torque [Nm]/1 -> Torque Limiter (outside) 2/1
  Inverse Gear Ratio2/1 -> Inverse Gear Ratio4/1
  Rotor and Gearing/3(Rotor Velocity [rad/s]) -> Rotor Damping/1
  Torque Limiter (outside) 2/1 -> Inverse Gear Ratio2/1
  connections:
  Rotor and Gearing/LConn1 -- Rotor Joint Conn/RConn1
